simulink model "modulation_assignment"  (R2021a)
settings: Solver=VariableStepDiscrete  StartTime=0.0  StopTime=0.02  RelTol=1e-3  EnableMultiTasking=on
InitFcn:
  | commpassbandmodParams.Fc = 2.5e6;
  | commpassbandmodParams.F1 = commpassbandmodParams.Fc/3+.5e5;
libraries: commutil2 x2, dspsrcs4 x2, commdigbbndpm3 x2, commfilt2 x2, commchan3 x1, commsink2 x1, commrandsrc3 x1
Description:
  | Passband Modulation
  | 
  | This model shows a straightforward way to perform passband modulation, by multiplying a modulated complex signal with a complex sine wave to perform frequency upconversion.
settings Model: Creator=The MathWorks, Inc.  LastModifiedBy=hewas
settings SolverCC: AlgebraicLoopSolver=TrustRegion  InsertRTBMode=Auto
settings DataIOCC: LimitDataPoints=on  SaveFormat=Array  SaveOutput=off  SignalLogging=off  SaveTime=off  ReturnWorkspaceOutputs=off
settings OptimizationCC: ExpressionDepthLimit=2147483647  InitFltsAndDblsToZero=on  EfficientMapNaN2IntZero=off  LifeSpan=inf
settings DebuggingCC: UnderspecifiedInitializationDetection=Classic  MergeDetectMultiDrivingBlocksExec=none  SolverPrmCheckMsg=warning  FcnCallInpInsideContextMsg=warning  AllowSymbolicDim=off  StateNameClashWarn=warning  SFUnexpectedBacktrackingDiag=warning  SFNoUnconditionalDefaultTransitionDiag=warning  SFExecutionAtInitializationDiag=none  SFMachineParentedDataDiag=warning  ArithmeticOperatorsInVariantConditions=warning
settings HardwareCC: ProdBitPerPointer=32  ProdBitPerSizeT=32  ProdBitPerPtrDiffT=32  ProdLargestAtomicFloat=None  ProdIntDivRoundTo=Undefined  ProdEndianess=Unspecified  ProdWordSize=32  ProdHWDeviceType=32-bit Generic
settings ModelReferenceCC: PropagateSignalLabelsOutOfModel=off
settings SFSimCC: SimUseLocalCustomCode=off  CustomCodeUndefinedFunction=UseInterfaceOnly
settings RTWCC: RTWUseLocalCustomCode=off
settings CodeAppCC: StateflowObjectComments=on
settings GRTTargetCC: TargetLangStandard=C89/C90 (ANSI)  CombineOutputUpdateFcns=off  GRTInterface=on
settings ConfigComp: CovMetricSettings=dw  CovSaveCumulativeToWorkspaceVar=on  CovSaveSingleToWorkspaceVar=on  CovExternalEMLEnable=off  CovSFcnEnable=off

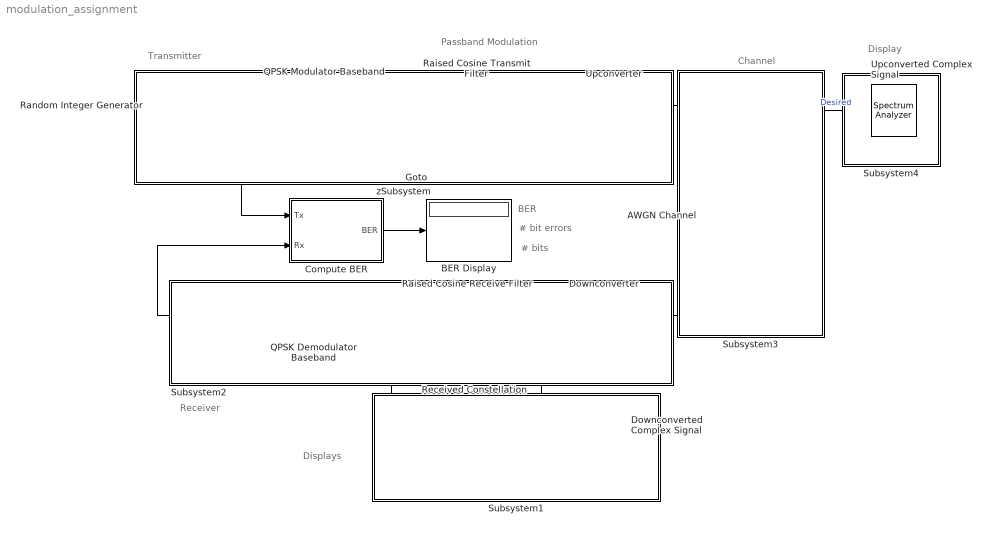
== system modulation_assignment ==
  note: Passband Modulation
  note: Transmitter
  note: Receiver
  note: Channel
  note: Displays
  note: Display
  note: BER
  note: # bit errors
  note: # bits
  AWGN Channel : commchan3/AWGN Channel  InputProcessing=Columns as channels (frame based)  seed=67  noiseMode="Signal to noise ratio  (Eb/No)"  EbNodB=8  EsNodB=10  SNRdB=10  bitsPerSym=2  Ps=1/(2*8)  Tsym=1e-6  variance=1
  BER Display : Display
  Compute BER : Subsystem
  Downconverted Complex Signal : SpectrumAnalyzer
  Downconverter : Subsystem
      mask Display: disp('Downconverter')
  QPSK Demodulator Baseband : commdigbbndpm3/QPSK Demodulator Baseband  OutType=Integer  DecType=Hard decision  VarSource=Dialog  Variance=1  Dec=Gray  Ph=pi/4  outDtype1=Inherit via internal rule  outDtype2=Inherit via internal rule  derotateFactorWordLen=16  derotateFactorDataTypeStr=Inherit: Same word length as input  derotateFactorLastDataTypeStr=Inherit: Same word length as input
  QPSK Modulator Baseband : commdigbbndpm3/QPSK Modulator Baseband  InType=Integer  Enc=Gray  Ph=pi/4  outDtype=double  outWordLen=16  outUDDataType=sfix(16)  outFracLenMode=Best precision  outFracLen=15  outDataTypeStr=double  outLastDataTypeStr=double
  Raised Cosine Receive Filter : commfilt2/Raised Cosine Receive Filter  filtType=Square root  R=0.2  filtSpan=8  N=8  downFactor=8  downOffset=0  filterGain=2  InputProcessing=Columns as channels (frame based)  RateOptions=Enforce single-rate processing  framing=Mute  checkCoeff=off  variableName=rcRxFilt1  currentFiltSpan=2*(4)  D=4  inputOffset=0  sampMode=Mute  saveAsFlag=0  rateMode=Downsampling  checkGain=User-specified  launchFVT=off  roundingMode=Floor  overflowMode=off  coeffDataTypeStr=Inherit: Same word length as input  coeffMin=[]  coeffMax=[]  coeffLastDataTypeStr=Inherit: Same word length as input  accumDataTypeStr=Inherit: Same as product output  accumLastDataTypeStr=Inherit: Same as product output  outputDataTypeStr=Inherit: Same as accumulator  outputMin=[]  outputMax=[]  outputLastDataTypeStr=Inherit: Same as accumulator
  Raised Cosine Transmit Filter : commfilt2/Raised Cosine Transmit Filter  filtType=Square root  R=0.2  filtSpan=8  N=8  filterGain=1  InputProcessing=Columns as channels (frame based)  RateOptions=Enforce single-rate processing  framing=Mute  checkCoeff=off  variableName=rcTxFilt1  checkGain=Normalized  sampMode=Mute  saveAsFlag=0  currentFiltSpan=2*(4)  D=4  launchFVT=off  roundingMode=Floor  overflowMode=off  coeffDataTypeStr=Inherit: Same word length as input  coeffMin=[]  coeffMax=[]  coeffLastDataTypeStr=Inherit: Same word length as input  outputDataTypeStr=Inherit: Same as accumulator  outputMin=[]  outputMax=[]  outputLastDataTypeStr=Inherit: Same as accumulator
  Random Integer Generator : commrandsrc3/Random Integer Generator  SetSize=4  SeedSource=Parameter  Seed=37  SampleTime=1e-6  SamplesPerFrame=100  OutputDataType=double  SimulateUsing=Interpreted execution
  Received Constellation : ConstellationDiagram  Tag=ScatterPlot
  Subsystem1 : Subsystem
      mask Display: disp('')
  Subsystem2 : Subsystem
      mask Display: disp('')
  Subsystem3 : Subsystem
      mask Display: disp('')
  Subsystem4 : Subsystem
      mask Display: disp('')
  Upconverted Complex Signal : SpectrumAnalyzer
  Upconverter : Subsystem
      mask Display: disp('Upconverter')
  zSubsystem : Subsystem
      mask Display: disp('')
  tag scope: TxSym=global
  wires:
  Random Integer Generator/1 -> QPSK Modulator Baseband/1, Compute BER/1(Tx)
  QPSK Modulator Baseband/1 -> Raised Cosine Transmit Filter/1, [TxSym]
  Compute BER/1(BER) -> BER Display/1
  QPSK Demodulator Baseband/1 -> Compute BER/2(Rx)
  AWGN Channel/1 -> Downconverter/1(In)
  Raised Cosine Transmit Filter/1 -> Upconverter/1(In)
  Raised Cosine Receive Filter/1 -> QPSK Demodulator Baseband/1, Received Constellation/1
  Downconverter/1(Out) -> Raised Cosine Receive Filter/1, Downconverted Complex Signal/1
  Upconverter/1(Out) -> AWGN Channel/1, Upconverted Complex Signal/1  "Desired"

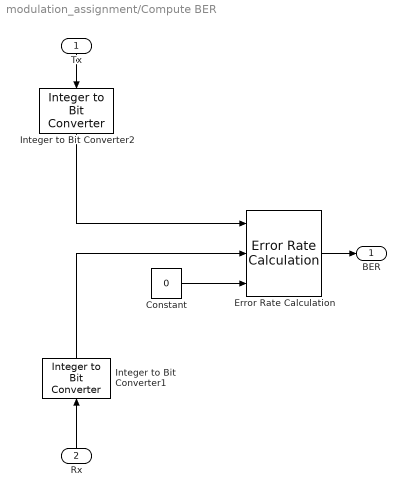
== system modulation_assignment/Compute BER ==
  Tx : Inport
  Rx : Inport  Port=2
  Constant : Constant  Value=0  SampleTime=1e-4
  Error Rate Calculation : commsink2/Error Rate Calculation  N=16  st_delay=0  cp_mode=Entire frame  subframe=[]  PMode=Port  WsName=ErrorVec  RsMode2=on  stop=off  numErr=100  maxBits=1e6
  Integer to Bit Converter1 : commutil2/Integer to Bit Converter  nbits=2  signedInputValues=Unsigned  bitOrder=MSB first  outDtype=boolean
  Integer to Bit Converter2 : commutil2/Integer to Bit Converter  nbits=2  signedInputValues=Unsigned  bitOrder=MSB first  outDtype=boolean
  BER : Outport  VectorParamsAs1DForOutWhenUnconnected=off
  wires:
  Integer to Bit Converter2/1 -> Error Rate Calculation/1
  Integer to Bit Converter1/1 -> Error Rate Calculation/2
  Tx/1 -> Integer to Bit Converter2/1
  Error Rate Calculation/1 -> BER/1
  Rx/1 -> Integer to Bit Converter1/1
  Constant/1 -> Error Rate Calculation/3

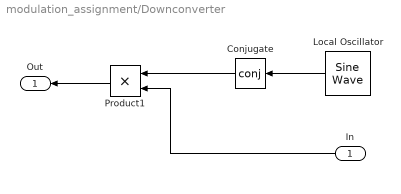
== system modulation_assignment/Downconverter ==
  In : Inport
  Conjugate : Math  Operator=conj  SignedPower=on  SaturateOnIntegerOverflow=on
  Local Oscillator : dspsrcs4/Sine Wave  Amplitude=1  Frequency=1000000  Phase=0  SampleMode=Discrete  OutComplex=Complex  CompMethod=Trigonometric fcn  TableSize=Speed  SampleTime=(1e-6) /8  SamplesPerFrame=800  ResetState=Restart at time zero  OutputFrames=off  dataType=double  wordLen=16  udDataType=sfix(16)  fracBitsMode=Best precision  numFracBits=15  OutDataTypeStr=double  LastOutDataTypeStr=double
  Product1 : Product  RndMeth=Zero
  Out : Outport  VectorParamsAs1DForOutWhenUnconnected=off
  wires:
  Conjugate/1 -> Product1/1
  Product1/1 -> Out/1
  In/1 -> Product1/2
  Local Oscillator/1 -> Conjugate/1

== system modulation_assignment/Subsystem1 ==

== system modulation_assignment/Subsystem2 ==

== system modulation_assignment/Subsystem3 ==

== system modulation_assignment/Subsystem4 ==

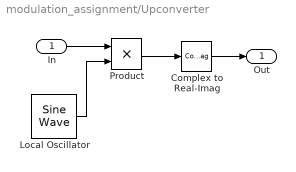
== system modulation_assignment/Upconverter ==
  In : Inport
  Complex to Real-Imag : ComplexToRealImag  Output=Real
  Local Oscillator : dspsrcs4/Sine Wave  Amplitude=1  Frequency=1000000  Phase=0  SampleMode=Discrete  OutComplex=Complex  CompMethod=Trigonometric fcn  TableSize=Speed  SampleTime=(1e-6) /8  SamplesPerFrame=800  ResetState=Restart at time zero  OutputFrames=off  dataType=double  wordLen=16  udDataType=sfix(16)  fracBitsMode=Best precision  numFracBits=15  OutDataTypeStr=double  LastOutDataTypeStr=double
  Product : Product  RndMeth=Zero
  Out : Outport  VectorParamsAs1DForOutWhenUnconnected=off
  wires:
  Complex to Real-Imag/1 -> Out/1
  Product/1 -> Complex to Real-Imag/1
  Local Oscillator/1 -> Product/2
  In/1 -> Product/1

== system modulation_assignment/zSubsystem ==
